simulink library "thermochemical"  (R2017b)
settings: Solver=VariableStepAuto  StartTime=0.0  StopTime=10.0  RelTol=1e-3
values from neighbouring files (symbols this model uses):
  c = conversion_factors()    [blk_clausius_clapeyron.m]    (also in blk_clausius_clapeyron_no_popup.m; blk_cold_room_closed_dry_air.m; blk_reactor_BaCl2_NH3_no_walls.m; blk_reactor_BaCl2_NH3_no_walls_state_space.m)
  cp = metal.cp    [blk_wall_simple.m]    (also in get_metal_properties.m = 390)
  fluid = get_param(blk,'fluid')    [blk_thermodynamic_properties_nonsaturated.m]    (also in blk_thermodynamic_properties_nonsaturated_interpreted.m; blk_thermodynamic_properties_saturated.m; blk_thermodynamic_properties_saturated_interpreted.m; blk_thermodynamic_properties_saturated_mix.m)
  gas = get_material_properties(x.gasName)    [blk_reactor_BaCl2_NH3_cylindrical_no_walls_fun1.m]
  h = get_param(gcb,'ObjectParameters')    [get_param_eval.m]
  rho = metal.rho    [blk_wall_simple.m]    (also in get_metal_properties.m = 8940)
  s = solve(eq,dx,'ReturnConditions',true)    [LMTD_inv.m]    (also in blk_wall_simple.m = get_param_eval(blk,'s'))
  u_gas_at_T_ref = -R * T_ref    [blk_reactor_BaCl2_NH3_no_walls.m]    (also in blk_reactor_BaCl2_NH3_no_walls_state_space.m)
undefined symbols (not defined in the file or in its folder): b_motor, BaCl2, beta, CoolProp, cP_binder, cP_gas, cP_s0, cv, dh_r_0, ENG, heat_exchanger_epsilonNTU_inv_simulink, heat_exchanger_epsilonNTU_simulink, J_motor, K_cin, kappa, Km_motor, La_motor, lookup2D_BreakPoint2, M_binder, N_binder, N_gas_free_volume_init, N_salt, NH3, nh3_v3, nu, P, phase, PID_D_motor, PID_I_motor, PID_P_motor, Ra_motor, Reactor_phase, T, T1, T2, T_init, Tr_init, Tr_ref, U_binder_at_Tr_ref, U_salt_at_X0_Tr_ref, Ur_init, V_void, Valve_regime, Vmax_motor, w_init_motor, X_init
libraries: thermochemical x247, simulink x54, dspsigops x3
(part 1 of 12)
settings Model: Creator=ferru  LastModifiedBy=fferrucc

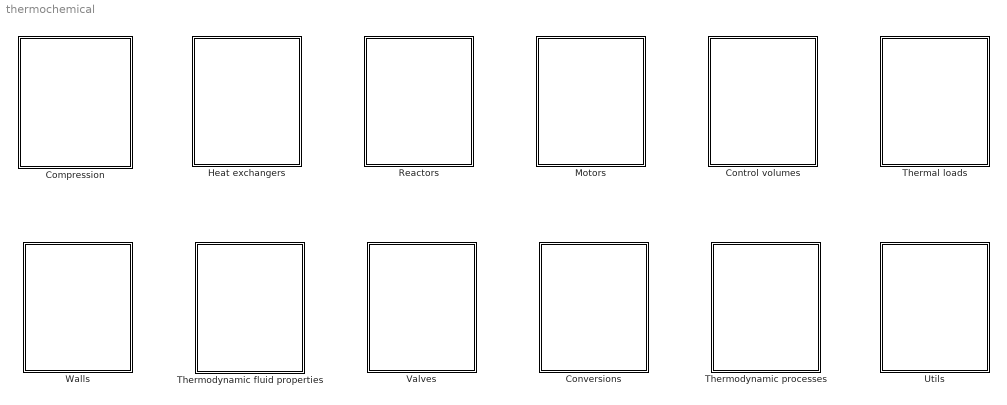
== system thermochemical ==
  Compression : Subsystem
  Control volumes : Subsystem
  Conversions : Subsystem
  Heat exchangers : Subsystem
  Motors : Subsystem
  Reactors : Subsystem
  Thermal loads : Subsystem
  Thermodynamic fluid properties : Subsystem
  Thermodynamic processes : Subsystem
  Utils : Subsystem
  Valves : Subsystem
  Walls : Subsystem

== system thermochemical/Compression ==
  Gas compressor without motor : Subsystem  mask{fluid=fluid, eta_IS=0.7, CL=0.03, eta_mech=0.9, dVswept_m3_h=6, dVswept_rmp=1500}
      mask prompts: fluid "Fluid properties (structure data type)"; eta_IS "Isentropic efficiency ([0..1])"; CL "Cylinder clearance ([0..1])"; eta_mech "Mechanical efficiency (compressor without motor) ([0..1])"; dVswept_m3_h "Swept volume rate at nominal speed (m³/h)"; dVswept_rmp "Nominal speed (rpm)"
      mask init:
      | % bar to Pascal conversion:
      | bar_to_Pa = 1e5;
  "Gas compressor without motor, two stages, ideal compression ratios" : Subsystem  mask{fluid=fluid, eta_IS=0.7, CL=0.03, eta_mech=0.9, dVswept_m3_h=6, dVswept_rmp=1500}
      mask prompts: fluid "Fluid properties (structure data type)"; eta_IS "Isentropic efficiency ([0..1])"; CL "Cylinder clearance ([0..1])"; eta_mech "Mechanical efficiency (compressor without motor) ([0..1])"; dVswept_m3_h "Swept volume rate at nominal speed (m³/h)"; dVswept_rmp "Nominal speed (rpm)"
      mask init:
      | % bar to Pascal conversion:
      | bar_to_Pa = 1e5;
  Irreversible compression process : Subsystem  mask(compression_irrev){fluid=fluid}
      mask prompts: fluid "Thermodynamic properties data (struct variable)"
      mask help: Irreversible compression process.
  Volumetric efficiency : Subsystem  mask(compression_volumetric_efficiency){}
      mask help:
      | Volumetric efficiency of a compression process.
      |
      | Ref: COMPRESSOR HANDBOOK, Paul C. Hanlon (editor), McGRAW-HILL, ISBN 0-07-026005-2, Sec. 1.2.5, page 1.11

== system thermochemical/Control volumes ==
  "Two-phase saturated fluid control volume (with wall, simple)" : Subsystem
  "Two-phase saturated fluid control volume (with wall, simple) (without algebraic loop)" : Subsystem
  "Two-phase saturated fluid control volume (with wall, tube with/without fins)" : Subsystem
  "Two-phase saturated fluid control volume (with wall, tube with/without fins) (without algebraic loop)" : Subsystem
  Two-phase saturated fluid control volume (without walls) : Subsystem  mask(volume_control_saturated){N_init=100, T_init=300, fluid=fluid, V=0.01}
      mask prompts: N_init "Initial number of mols inside the control volume (mol)"; T_init "Fluid initial temperature (K)"; fluid "Fluid (structure data type)"; V "Volume (m3)"
      mask help:
      | This block models a volume control that contains a fluid always in its saturation state.
      |
      | The model can work as a condenser or as an evaporator:
      | • Condenser: connect the output 'h liq (J/mol)' to the input 'h out (sat) (J/mol)'
      | • Evaporator: connect the output 'h vap (J/mol)' to the input 'h out (sat) (J/mol)'
      |
      | The ratio between the two phases is given by two outputs:
      | 1) volumetric liquid fraction: liquid volume/total volume (0..1)
      | 2) vapor quality (e.g. zero: 100% liquid, one: 100% vapor).
      |
      | Note 2: the model is not prepared to work in the non-saturation state of the fluid (e.g. superheated gas or supercooled liquid). This means that both the liquid fraction and the vapor quality are strictly constrained in the (0..1) open range. The simulation will stop if these constrains are violated.
      mask DialogControl Container3 Prompt: Initial state
      mask DialogControl Container4 Prompt: Other parameters
  Two-phase saturated fluid control volume (without walls) (without algebraic loop) : Subsystem  mask(volume_control_saturated){N_init=100, T_init=300, fluid=fluid, V=0.01}
      mask prompts: N_init "Initial number of mols inside the control volume (mol)"; T_init "Fluid initial temperature (K)"; fluid "Fluid (structure data type)"; V "Volume (m3)"
      mask help:
      | This block models a volume control that contains a fluid always in its saturation state.
      |
      | The model can work as a condenser or as an evaporator:
      | • Condenser: connect the output 'h liq (J/mol)' to the input 'h out (sat) (J/mol)'
      | • Evaporator: connect the output 'h vap (J/mol)' to the input 'h out (sat) (J/mol)'
      |
      | The ratio between the two phases is given by two outputs:
      | 1) volumetric liquid fraction: liquid volume/total volume (0..1)
      | 2) vapor quality (e.g. zero: 100% liquid, one: 100% vapor).
      |
      | Note 2: the model is not prepared to work in the non-saturation state of the fluid (e.g. superheated gas or supercooled liquid). This means that both the liquid fraction and the vapor quality are strictly constrained in the (0..1) open range. The simulation will stop if these constrains are violated.
      mask init:
      | c = conversion_factors();
      mask DialogControl Container3 Prompt: Initial state
      mask DialogControl Container4 Prompt: Other parameters
  Two-phase saturated fluid control volume energy equation : Subsystem  mask(control_volume_energy_equation){fluid=fluid}
      mask prompts: fluid "Fluid (structure data type)"
  "Two-phase saturated fluid control volume (with wall, simple) + heat exchanger (condensation/evaporation), with water loop" : Subsystem
  "Two-phase saturated fluid control volume (with wall, simple) + heat exchanger (condensation/evaporation), with water loop (without algebraic loop)" : Subsystem

== system thermochemical/Conversions ==
  Pressure conversion : Subsystem  mask(convert_pressure){sel=Pa --> bar}
      mask prompts: sel "Conversion"
      mask help: Conversion between pressure units.
      mask init:
      | % Get mask parameters:
      | blk = gcb;
      | par = get_param(blk,'sel');
      | c = conversion_factors();
      | switch par
      | %-----------------
      |     case 'Pa --> bar'
      |         in1    = '(Pa)';
      |         out1   = '(bar)';
      |         K = c.Pa_to_bar;
      |     case 'Pa --> kPa'
      |         in1    = '(Pa)';
      |         out1   = '(kPa)';
      |         K = c.Pa_to_kPa;
      |     case 'Pa --> psi'
      |         in1   = '(Pa)';
      |         out1  = '(psi)';
      |         K = c.Pa_to_psi;
      |     case 'Pa --> atm'
      |         in1    = '(Pa)';
      |         out1   = '(atm)';
      |         K = c.Pa_to_atm;
      | %-----------------
      |     case 'kPa --> bar'
      |         in1    = '(kPa)';
      |         out1   = '(bar)';
      |         K = c.kPa_to_bar;
      |     case 'kPa --> Pa'
      |         in1    = '(kPa)';
      |         out1   = '(Pa)';
      |         K = c.kPa_to_Pa;
      |     case 'kPa --> psi'
      |         in1   = '(kPa)';
      |         out1  = '(psi)';
      |         K = c.kPa_to_psi;
      |     case 'kPa --> atm'
      |         in1    = '(kPa)';
      |         out1   = '(atm)';
      |         K = c.kPa_to_atm;
      | %-----------------
      |     case 'bar --> Pa'
      |         in1    = '(bar)';
      |         out1   = '(Pa)';
      |         K = c.bar_to_Pa;
      |     case 'bar --> kPa'
      |         in1    = '(bar)';
      |         out1   = '(kPa)';
      |         K = c.bar_to_kPa;
      |     case 'bar --> psi'
      |         in1   = '(bar)';
      |         out1  = '(psi)';
      |         K = c.bar_to_psi;
      |     case 'bar --> atm'
      |         in1    = '(bar)';
      |         out1   = '(atm)';
      |         K = c.bar_to_atm;
      | %-----------------      
      |     case 'psi --> bar'
      |         in1   = '(psi)';
      |         out1  = '(bar)';
      |         K = c.psi_to_bar;
      |     case 'psi --> Pa'
      |         in1    = '(psi)';
      |         out1   = '(Pa)';
      |         K = c.psi_to_Pa;
      |     case 'psi --> kPa'
      |         in1    = '(psi)';
      |         out1   = '(kPa)';
      |         K = c.psi_to_kPa;
      |     case 'psi --> atm'
      |         in1    = '(psi)';
      |         out1   = '(atm)';
      |         K = c.psi_to_atm;
      | %-----------------
      |     case 'atm --> bar'
      |         in1   = '(atm)';
      |         out1  = '(bar)';
      |         K = c.atm_to_bar;
      |     case 'atm --> Pa'
      |         in1    = '(atm)';
      |         out1   = '(Pa)';
      |         K = c.atm_to_Pa;
      |     case 'atm --> kPa'
      |         in1    = '(atm)';
      |         out1   = '(kPa)';
      |         K = c.atm_to_kPa;
      |     case 'atm --> psi'
      |         in1   = '(atm)';
      |         out1  = '(psi)';
      |         K = c.atm_to_psi;
      | %-----------------
      | end
      | 
      | % % Set mask parameters:
      | set_param([blk,'/Gain'],'Gain',num2str(K))
      | % 
      | % % Change name of input 1:
      | p = get_param([blk,'/In1'],'PortHandles');
      | q = get_param(p.Outport,'Line');
      | set_param(q,'Name',in1);
      | % 
      | % % Change name of output:
      | p = get_param([blk,'/Out1'],'PortHandles');
      | q = get_param(p.Inport,'Line');
      | set_param(q,'Name',out1);
      mask TypeOptions sel: Pa --> bar | Pa --> kPa | Pa --> psi | Pa --> atm | kPa --> bar | kPa --> Pa | kPa --> psi | kPa --> atm | bar --> Pa | bar --> kPa | bar --> psi | bar --> atm | psi --> bar | psi --> Pa | psi --> kPa | psi --> atm | atm --> bar | atm --> Pa | atm --> kPa | atm --> psi
  Rotational speed conversion : Subsystem  mask(convert_pressure){sel=rpm --> rad/sec}
      mask prompts: sel "Conversion"
      mask help: Conversion between pressure units.
      mask init:
      | % Get mask parameters:
      | blk = gcb;
      | par = get_param(blk,'sel');
      | c = conversion_factors();
      | 
      | switch par
      | %-----------------
      |     case 'rpm --> rad/sec'
      |         in1    = '(rpm)';
      |         out1   = '(rad/sec)';
      |         K = c.rpm_to_rad_sec;
      |     case 'rpm --> rev/sec'
      |         in1    = '(rpm)';
      |         out1   = '(rev/sec)';
      |         K = c.rpm_to_rev_sec;
      |     case 'rad/sec --> rpm'
      |         in1   = '(rad/sec)';
      |         out1  = '(rpm)';
      |         K = c.rad_sec_to_rpm;
      |     case 'rad/sec --> rev/sec'
      |         in1    = '(rad/sec)';
      |         out1   = '(rev/sec)';
      |         K = c.rad_sec_to_rev_sec;
      |     case 'rev/sec --> rpm'
      |         in1    = '(rev/sec)';
      |         out1   = '(rpm)';
      |         K = c.rev_sec_to_rpm;
      |     case 'rev/sec --> rad/sec'
      |         in1    = '(rev/sec)';
      |         out1   = '(rad/sec)';
      |         K = c.rev_sec_to_rad_sec;
      |     otherwise
      |         error('It shouldn''t have gotten in her!')
      | end
      | 
      | % % Set mask parameters:
      | set_param([blk,'/Gain'],'Gain',num2str(K))
      | % 
      | % % Change name of input 1:
      | p = get_param([blk,'/In1'],'PortHandles');
      | q = get_param(p.Outport,'Line');
      | set_param(q,'Name',in1);
      | % 
      | % % Change name of output:
      | p = get_param([blk,'/Out1'],'PortHandles');
      | q = get_param(p.Inport,'Line');
      | set_param(q,'Name',out1);
      mask TypeOptions sel: rpm --> rad/sec | rpm --> rev/sec | rad/sec --> rpm | rad/sec --> rev/sec | rev/sec --> rpm | rev/sec --> rad/sec
  Temperature conversion : Subsystem  mask(convert_temperature){sel=°R --> °F}
      mask prompts: sel "Conversion"
      mask help: Conversion between temperature units.
      mask init:
      | % Get mask parameters:
      | blk = gcb;
      | par = get_param(blk,'sel');
      | 
      | switch par
      |     case 'K --> °C'
      |         in1   = '(K)';
      |         out1  = '(°C)';
      |         count = 1;
      |     case '°C --> K'
      |         in1   = '(°C)';
      |         out1  = '(K)';
      |         count = 2;
      |     case '°C --> °F'
      |         in1   = '(°C)';
      |         out1  = '(°F)';
      |         count = 3;  
      |     case '°F --> °C'
      |         in1    = '(°F)';
      |         out1   = '(°C)';
      |         count = 4;     
      |     case 'K --> °F'
      |         in1   = '(K)';
      |         out1  = '(°F)';
      |         count = 5;
      |     case '°F --> K'
      |         in1    = '(°F)';
      |         out1  = '(K)';
      |         count = 6;
      |     case '°R --> °C'
      |         in1   = '(°R)';
      |         out1  = '(°C)';
      |         count = 7;
      |     case '°C --> °R'
      |         in1   = '(°C)';
      |         out1  = '(°R)';
      |         count = 8;
      |     case '°R --> °F'
      |         in1   = '(°R)';
      |         out1  = '(°F)';
      |         count = 9;  
      |     case '°F --> °R'
      |         in1    = '(°F)';
      |         out1   = '(°R)';
      |         count = 10;
      |     case 'K --> °R'
      |         in1   = '(K)';
      |         out1  = '(°R)';
      |         count = 11;
      |     case '°R --> K'
      |         in1    = '(°R)';
      |         out1  = '(K)';
      |         count = 12;
      | end
      | 
      | % Set mask parameters:
      | set_param([blk,'/Constant'],'Value',num2str(count))
      | 
      | % Change name of input 1:
      | p = get_param([blk,'/In1'],'PortHandles');
      | q = get_param(p.Outport,'Line');
      | set_param(q,'Name',in1);
      | 
      | % Change name of output:
      | p = get_param([blk,'/Out1'],'PortHandles');
      | q = get_param(p.Inport,'Line');
      | set_param(q,'Name',out1);
      mask TypeOptions sel: K --> °C | K --> °F | K --> °R | °C --> K | °C --> °F | °C --> °R | °F --> K | °F --> °C | °F --> °R | °R --> K | °R --> °C | °R --> °F
  Volume flow rate conversion : Subsystem  mask(convert_volume_flow){sel=m3/h --> CFM}
      mask prompts: sel "Conversion"
      mask help: Conversion between volume flow rate units.
      mask init:
      | % Get mask parameters:
      | blk = gcb;
      | par = get_param(blk,'sel');
      | c = conversion_factors();
      | 
      | switch par
      |     case 'm3/sec --> m3/h'
      |         in1    = '(m3/sec)';
      |         out1   = '(m3/h)';    
      |         K      = c.m3_sec_to_m3_h;
      |     case 'm3/sec --> L/min'
      |         in1    = '(m3/sec)';
      |         out1   = '(L/min)';    
      |         K      = c.m3_sec_to_L_min;
      |     case 'm3/sec --> gpmUS'
      |         in1    = '(m3/sec)';
      |         out1   = '(gpmUS)';    
      |         K      = c.m3_sec_to_gpmUS;
      |     case 'm3/sec --> CFH'
      |         in1    = '(m3/sec)';
      |         out1   = '(CFH)';    
      |         K      = c.m3_sec_to_CFH;
      |     case 'm3/sec --> CFM'
      |         in1    = '(m3/sec)';
      |         out1   = '(CFM)';    
      |         K      = c.m3_sec_to_CFM;
      |     case 'L/min --> m3/sec'
      |         in1    = '(L/min)';
      |         out1   = '(m3/sec)';    
      |         K      = c.L_min_to_m3_sec;
      |     case 'L/min --> m3/h'
      |         in1    = '(L/min)';
      |         out1   = '(m3/h)';    
      |         K      = c.L_min_to_m3_h;
      |     case 'L/min --> gpmUS'
      |         in1    = '(L/min)';
      |         out1   = '(gpmUS)';    
      |         K      = c.L_min_to_gpmUS;
      |     case 'L/min --> CFH'
      |         in1    = '(L/min)';
      |         out1   = '(CFH)';    
      |         K      = c.L_min_to_CFH;
      |     case 'L/min --> CFM'
      |         in1    = '(L/min)';
      |         out1   = '(CFM)';    
      |         K      = c.L_min_to_CFM;
      |     case 'm3/h --> m3/sec'
      |         in1    = '(m3/h)';
      |         out1   = '(m3/sec)';    
      |         K      = c.m3_h_to_m3_sec;
      |     case 'm3/h --> L/min'
      |         in1    = '(m3/h)';
      |         out1   = '(L/min)';    
      |         K      = c.m3_h_to_L_min;
      |     case 'm3/h --> gpmUS'
      |         in1    = '(m3/h)';
      |         out1   = '(gpmUS)';    
      |         K      = c.m3_h_to_gpmUS;
      |     case 'm3/h --> CFH'
      |         in1    = '(m3/h)';
      |         out1   = '(CFH)';    
      |         K      = c.m3_h_to_CFH;
      |     case 'm3/h --> CFM'
      |         in1    = '(m3/h)';
      |         out1   = '(CFM)';    
      |         K      = c.m3_h_to_CFM;
      |     case 'gpmUS --> m3/sec'
      |         in1    = '(gpmUS)';
      |         out1   = '(m3/sec)';    
      |         K      = c.gpmUS_to_m3_sec;
      |     case 'gpmUS --> m3/h'
      |         in1    = '(gpmUS)';
      |         out1   = '(m3/h)';    
      |         K      = c.gpmUS_to_m3_h;
      |     case 'gpmUS --> L/min'
      |         in1    = '(gpmUS)';
      |         out1   = '(L/min)';    
      |         K      = c.gpmUS_to_L_min;
      |     case 'gpmUS --> CFH'
      |         in1    = '(gpmUS)';
      |         out1   = '(CFH)';    
      |         K      = c.gpmUS_to_CFH;
      |     case 'gpmUS --> CFM'
      |         in1    = '(gpmUS)';
      |         out1   = '(CFM)';    
      |         K      = c.gpmUS_to_CFM;
      |     case 'CFH --> m3/sec'
      |         in1    = '(CFH)';
      |         out1   = '(m3/sec)';    
      |         K      = c.CFH_to_m3_sec;
      |     case 'CFH --> m3/h'
      |         in1    = '(CFH)';
      |         out1   = '(m3/h)';    
      |         K      = c.CFH_to_m3_h;
      |     case 'CFH --> L/min'
      |         in1    = '(CFH)';
      |         out1   = '(L/min)';    
      |         K      = c.CFH_to_L_min;
      |     case 'CFH --> gpmUS'
      |         in1    = '(CFH)';
      |         out1   = '(gpmUS)';    
      |         K      = c.CFH_to_gpmUS;
      |     case 'CFH --> CFM'
      |         in1    = '(CFH)';
      |         out1   = '(CFM)';    
      |         K      = c.CFH_to_CFM;
      |     case 'CFM --> m3/sec'
      |         in1    = '(CFM)';
      |         out1   = '(m3/sec)';    
      |         K      = c.CFM_to_m3_sec;
      |     case 'CFM --> m3/h'
      |         in1    = '(CFM)';
      |         out1   = '(m3/h)';    
      |         K      = c.CFM_to_m3_h;
      |     case 'CFM --> L/min'
      |         in1    = '(CFM)';
      |         out1   = '(L/min)';    
      |         K      = c.CFM_to_L_min;
      |     case 'CFM --> gpmUS'
      |         in1    = '(CFM)';
      |         out1   = '(gpmUS)';    
      |         K      = c.CFM_to_gpmUS;
      |     case 'CFM --> CFH'
      |         in1    = '(CFM)';
      |         out1   = '(CFH)';    
      |         K      = c.CFM_to_CFH;
      |     otherwise
      |         error('It shouldn''t have entered here!')
      | end
      | 
      | % Set mask parameters:
      | set_param([blk,'/Gain'],'Gain',num2str(K))
      |  
      | % Change name of input 1:
      | p = get_param([blk,'/In1'],'PortHandles');
      | q = get_param(p.Outport,'Line');
      | set_param(q,'Name',in1);
      |  
      | % Change name of output:
      | p = get_param([blk,'/Out1'],'PortHandles');
      | q = get_param(p.Inport,'Line');
      | set_param(q,'Name',out1);
      mask TypeOptions sel: m3/sec --> m3/h | m3/sec --> L/min | m3/sec --> gpmUS | m3/sec --> CFH | m3/sec --> CFM | L/min --> m3/sec | L/min --> m3/h | L/min --> gpmUS | L/min --> CFH | L/min --> CFM | m3/h --> m3/sec | m3/h --> L/min | m3/h --> gpmUS | m3/h --> CFH | m3/h --> CFM | gpmUS --> m3/sec | gpmUS --> m3/h | gpmUS --> L/min | gpmUS --> CFH | gpmUS --> CFM | CFH --> m3/sec | CFH --> m3/h | CFH --> L/min | CFH --> gpmUS | CFH --> CFM | CFM --> m3/sec | CFM --> m3/h | CFM --> L/min | CFM --> gpmUS | CFM --> CFH

== system thermochemical/Heat exchangers ==
  "Heat Exchanger, e-NTU method (UA input) (it uses CoolProp library)" : Subsystem  mask(heat_exchanger_eNTU){fluidName_1=Water, fluidName_2=Water, flowType=Counter-flow}
      mask prompts: fluidName_1 "Stream 1 fluid name (must be available in CoolProp library)"; fluidName_2 "Stream 2 fluid name (must be available in CoolProp library)"; flowType "Flow arrangement"
      mask help:
      | Heat Exchanger, e-NTU method.
      | The block assumes:
      | * null pressure drop in the streams
      | * steady state
      | The values of heat capacities are computed at an average temperature value between the inlet and outlet temperatures. The block uses the CoolProp library (see help for references).
      |
      | The dimensionless number Cr = d(Cmin)/dt / d(Cmax)/dt is the capacity ratio and reﬂects how well-balanced the heat exchanger is.
      | If the capacity ratio is unity, then the heat exchanger is operating in a balanced condition; the capacitance rates of the two ﬂuids and therefore the temperature change experienced by the two ﬂuids are the same. If the capacity ratio is very small, then the heat exchanger is operating in an unbalanced condition; the capacitance rate of one ﬂuid is very large compared to the other and the temperature of this ﬂuid will not change substantially. This situation occurs when one ﬂuid is changing phase.
      mask init:
      | % NOTE: Everything that is writen here will go to MaskInitialization parameter
      | 
      | % Get mask parameters:
      | blk = gcb;
      | fluidName_h = get_param(blk,'fluidName_1');
      | fluidName_c = get_param(blk,'fluidName_2');
      | flowType = get_param(blk,'flowType');
      | 
      | % Set value of Interpreted Matlab function according to menu's parameters:
      | str = ['heat_exchanger_epsilonNTU_simulink(u(1),u(2),u(3),''',fluidName_1,''',u(4),u(5),u(6),''',fluidName_2,''',u(7),''',flowType,''')'];
      | set_param([blk,'/heat_exchanger'],'MATLABFcn',str);
      | 
      | % Debug only:
      | % disp(str)
      mask Help:
      | Ref:
      | [1] Gregory Nellis, Sanford Klein -  Heat Transfer - Cambridge University Press (2008). Section 8.
      | [2] Ian H. Bell, Jorrit Wronski, Sylvain Quoilin, and Vincent Lemort,Pure and pseudo-pure fluid thermophysical  property evaluation  and  the  open-source  thermophysical  property  library  cool-prop, Industrial & Engineering Chemistry Research 53 (2014), no. 6, 2498–2508.
      mask TypeOptions flowType: Counter-flow | Parallel-flow | Cross-flow, both unmixed | Cross-flow, both mixed | Cross-flow, Cmax mixed, Cmin unmixed | Cross-flow, Cmin mixed, Cmax unmixed
  "Heat Exchanger, e-NTU method (UA input) Loop 2: water" : Subsystem  mask(heat_exchanger_eNTU_inv_2){fluid=fluid, flowType=Counter-flow, cp_water_J_K_mol=75.3260}
      mask prompts: fluid "Thermodynamic properties data for fluid 1 (struct variable)"; flowType "Flow arrangement"; cp_water_J_K_mol "Cp of water (J/K·mol)"
      mask help:
      | Heat Exchanger, e-NTU method (inverse)
      | The block accepts 'epsilon' as input and returns the conductance 'U*A' (W/K).
      | The block assumes:
      | * null pressure drop in the streams
      | * steady state
      | * loop 2 fluid is water
      | The values of heat capacity for fluid in loop 1 is computed at an average temperature value between the inlet and outlet temperatures.
      |
      | The dimensionless number Cr = d(Cmin)/dt / d(Cmax)/dt is the capacity ratio and reﬂects how well-balanced the heat exchanger is.
      | If the capacity ratio is unity, then the heat exchanger is operating in a balanced condition; the capacitance rates of the two ﬂuids and therefore the temperature change experienced by the two ﬂuids are the same. If the capacity ratio is very small, then the heat exchanger is operating in an unbalanced condition; the capacitance rate of one ﬂuid is very large compared to the other and the temperature of this ﬂuid will not change substantially. This situation occurs when one ﬂuid is changing phase.
      mask init:
      | % NOTE: Everything that is writen here will go to MaskInitialization parameter
      | 
      | % Get mask parameters:
      | blk = gcb;
      | flow = get_param(blk,'flowType');
      | 
      | % Compute 'flowType_numeric' according to 'flowType' dialog variable:
      | switch(flow)
      |     case 'Counter-flow'
      |         flowType_numeric = 0;
      |     case 'Parallel-flow'
      |         flowType_numeric = 1;
      |     case 'Cross-flow, both unmixed'
      |         flowType_numeric = 2;
      |     case 'Cross-flow, both mixed'
      |         flowType_numeric = 3;
      |     case 'Cross-flow, Cmax mixed, Cmin unmixed'
      |         flowType_numeric = 4;
      |     case 'Cross-flow, Cmin mixed, Cmax unmixed'
      |         flowType_numeric = 5;
      |     case 'Condensation/evaporation'
      |         flowType_numeric = 6;
      |     otherwise
      |         flowType_numeric = -1;
      |         error('Wrong flow type or flow type not implemented.')
      | end
      | 
      | % Set value of constant block:
      | set_param([blk,'/Subsystem/NTU as a function of flow configuration/Flow type (numeric)'],...
      |            'Value',num2str(flowType_numeric));
      mask Help:
      | Ref:
      | [1] Gregory Nellis, Sanford Klein -  Heat Transfer - Cambridge University Press (2008). Section 8.
      | [2] Ian H. Bell, Jorrit Wronski, Sylvain Quoilin, and Vincent Lemort,Pure and pseudo-pure fluid thermophysical  property evaluation  and  the  open-source  thermophysical  property  library  cool-prop, Industrial & Engineering Chemistry Research 53 (2014), no. 6, 2498–2508.
      mask TypeOptions flowType: Counter-flow | Parallel-flow | Cross-flow, both unmixed | Cross-flow, Cmax mixed, Cmin unmixed | Cross-flow, Cmin mixed, Cmax unmixed
  "Heat Exchanger, e-NTU method (UA input) One fluid or condensation/evaporation Loop 2: water" : Subsystem  mask(heat_exchanger_one_fluid_eNTU){cp_water_J_K_mol=75.3260}
      mask prompts: cp_water_J_K_mol "Cp of water (J/K·mol)"
      mask help:
      | Heat Exchanger, one-fluid configuration (isothermal wall), e-NTU method
      |
      | The block accepts the conductance 'U*A' (W/K) as input and returns 'epsilon'.
      |
      | The block assumes:
      | * null pressure drop in the water stream
      | * steady state
      | * loop 1 has constant temperature
      | * loop 2 fluid is water
      mask Help:
      | Ref:
      | [1] Gregory Nellis, Sanford Klein -  Heat Transfer - Cambridge University Press (2008). Section 8.
      | [2] Ian H. Bell, Jorrit Wronski, Sylvain Quoilin, and Vincent Lemort,Pure and pseudo-pure fluid thermophysical  property evaluation  and  the  open-source  thermophysical  property  library  cool-prop, Industrial & Engineering Chemistry Research 53 (2014), no. 6, 2498–2508.
  "Heat Exchanger, e-NTU method (epsilon input) (it uses CoolProp library)" : Subsystem  mask(heat_exchanger_eNTU_inv){fluidName_1=Water, fluidName_2=Water, flowType=Counter-flow}
      mask prompts: fluidName_1 "Stream 1 fluid name (must be available in CoolProp library)"; fluidName_2 "Stream 2 fluid name (must be available in CoolProp library)"; flowType "Flow arrangement"
      mask help:
      | Heat Exchanger, e-NTU method (inverse)
      | The block accepts 'epsilon' as input and returns the conductance 'U*A' (W/K).
      | The block assumes:
      | * null pressure drop in the streams
      | * steady state
      | The values of heat capacities are computed at an average temperature value between the inlet and outlet temperatures. The block uses the CoolProp library (see help for references).
      |
      | The dimensionless number Cr = d(Cmin)/dt / d(Cmax)/dt is the capacity ratio and reﬂects how well-balanced the heat exchanger is.
      | If the capacity ratio is unity, then the heat exchanger is operating in a balanced condition; the capacitance rates of the two ﬂuids and therefore the temperature change experienced by the two ﬂuids are the same. If the capacity ratio is very small, then the heat exchanger is operating in an unbalanced condition; the capacitance rate of one ﬂuid is very large compared to the other and the temperature of this ﬂuid will not change substantially. This situation occurs when one ﬂuid is changing phase.
      mask init:
      | % NOTE: Everything that is writen here will go to MaskInitialization parameter
      | 
      | % Get mask parameters:
      | blk = gcb;
      | fluidName_1 = get_param(blk,'fluidName_1');
      | fluidName_2 = get_param(blk,'fluidName_2');
      | flowType = get_param(blk,'flowType');
      | 
      | % Set value of Interpreted Matlab function according to menu's parameters:
      | str = ['heat_exchanger_epsilonNTU_inv_simulink(u(1),u(2),u(3),''',fluidName_1,''',u(4),u(5),u(6),''',fluidName_2,''',u(7),''',flowType,''')'];
      | set_param([blk,'/heat_exchanger'],'MATLABFcn',str);
      | 
      | % Debug only:
      | % disp(str)
      mask Help:
      | Ref:
      | [1] Gregory Nellis, Sanford Klein -  Heat Transfer - Cambridge University Press (2008). Section 8.
      | [2] Ian H. Bell, Jorrit Wronski, Sylvain Quoilin, and Vincent Lemort,Pure and pseudo-pure fluid thermophysical  property evaluation  and  the  open-source  thermophysical  property  library  cool-prop, Industrial & Engineering Chemistry Research 53 (2014), no. 6, 2498–2508.
      mask TypeOptions flowType: Counter-flow | Parallel-flow | Cross-flow, both unmixed | Cross-flow, Cmax mixed, Cmin unmixed | Cross-flow, Cmin mixed, Cmax unmixed
  "Heat Exchanger, e-NTU method (epsilon input) Loop 2: water" : Subsystem  mask(heat_exchanger_eNTU_inv_2){fluid=fluid, flowType=Counter-flow, cp_water_J_K_mol=75.3260}
      mask prompts: fluid "Thermodynamic properties data for fluid 1 (struct variable)"; flowType "Flow arrangement"; cp_water_J_K_mol "Cp of water (J/K·mol)"
      mask help:
      | Heat Exchanger, e-NTU method (inverse)
      | The block accepts 'epsilon' as input and returns the conductance 'U*A' (W/K).
      | The block assumes:
      | * null pressure drop in the streams
      | * steady state
      | * loop 2 fluid is water
      | The values of heat capacity for fluid in loop 1 is computed at an average temperature value between the inlet and outlet temperatures.
      |
      | The dimensionless number Cr = d(Cmin)/dt / d(Cmax)/dt is the capacity ratio and reﬂects how well-balanced the heat exchanger is.
      | If the capacity ratio is unity, then the heat exchanger is operating in a balanced condition; the capacitance rates of the two ﬂuids and therefore the temperature change experienced by the two ﬂuids are the same. If the capacity ratio is very small, then the heat exchanger is operating in an unbalanced condition; the capacitance rate of one ﬂuid is very large compared to the other and the temperature of this ﬂuid will not change substantially. This situation occurs when one ﬂuid is changing phase.
      mask init: same as thermochemical/Heat exchangers/Heat Exchanger, e-NTU method (UA input) Loop 2: water
      mask Help:
      | Ref:
      | [1] Gregory Nellis, Sanford Klein -  Heat Transfer - Cambridge University Press (2008). Section 8.
      | [2] Ian H. Bell, Jorrit Wronski, Sylvain Quoilin, and Vincent Lemort,Pure and pseudo-pure fluid thermophysical  property evaluation  and  the  open-source  thermophysical  property  library  cool-prop, Industrial & Engineering Chemistry Research 53 (2014), no. 6, 2498–2508.
      mask TypeOptions flowType: Counter-flow | Parallel-flow | Cross-flow, both unmixed | Cross-flow, Cmax mixed, Cmin unmixed | Cross-flow, Cmin mixed, Cmax unmixed
  "Heat Exchanger, e-NTU method (epsilon input) One fluid or condensation/evaporation Loop 2: water" : Subsystem  mask(heat_exchanger_one_fluid_eNTU_inv){cp_water_J_K_mol=75.3260}
      mask prompts: cp_water_J_K_mol "Cp of water (J/K·mol)"
      mask help:
      | Heat Exchanger, one-fluid configuration (isothermal wall), e-NTU method (inverse)
      |
      | The block accepts 'epsilon' as input and returns the conductance 'U*A' (W/K).
      |
      | The block assumes:
      | * null pressure drop in the water stream
      | * steady state
      | * loop 1 has constant temperature
      | * loop 2 fluid is water
      mask Help:
      | Ref:
      | [1] Gregory Nellis, Sanford Klein -  Heat Transfer - Cambridge University Press (2008). Section 8.
      | [2] Ian H. Bell, Jorrit Wronski, Sylvain Quoilin, and Vincent Lemort,Pure and pseudo-pure fluid thermophysical  property evaluation  and  the  open-source  thermophysical  property  library  cool-prop, Industrial & Engineering Chemistry Research 53 (2014), no. 6, 2498–2508.
  LMTD : Subsystem

== system thermochemical/Motors ==
  DC motor + DC power supply + speed controller : Subsystem  mask(dc_motor_plus_speed_controller_plus_DC_power_source){L=La_motor, R=Ra_motor, J=J_motor, b=b_motor, Km=Km_motor, w_init_motor=w_init_motor, PID_P=PID_P_motor, PID_I=PID_I_motor, PID_D=PID_D_motor, V_max=Vmax_motor}
      mask prompts: L "Armature inductance (Hy)"; R "Armature resistance (Ohm)"; J "Mechanical inertia (kg.m²)"; b "Viscous friction coefficient (N.m.sec)"; Km "Electromechanical constant (N.m/A)"; w_init_motor "Motor initial speed (rad/sec)"; PID_P "Proportional gain"; PID_I "Integral gain"; PID_D "Derivative gain"; V_max "Maximum output voltage (V)"
      mask DialogControl Container3 Prompt: DC motor
      mask DialogControl Container4 Prompt: Motor speed controller (PDI controller)
      mask DialogControl Container5 Prompt: Power source
  "DC motor, permanent magnet, one-way rotation" : Subsystem  mask(dc_motor_permanent_magnet_one_way_rotation){L=2.31e-3, R=0.83, J=0.1, b=2.5e-4, Km=1.3, w_init=0}
      mask prompts: L "Armature inductance (Hy)"; R "Armature resistance (Ohm)"; J "Mechanical inertia (kg.m²)"; b "Viscous friction coefficient (N.m.sec)"; Km "Electromechanical constant (N.m/A)"; w_init "Motor initial speed (rad/sec)"

== system thermochemical/Reactors ==
  Reactor's internal energy equation : Subsystem  mask(reactor_internal_energy){Tr_ref=Tr_ref, N_salt=N_salt, cP_s0=cP_s0, U_salt_at_X0_Tr_ref=U_salt_at_X0_Tr_ref, N_binder=N_binder, M_binder=M_binder, cP_binder=cP_binder, U_binder_at_Tr_ref=U_binder_at_Tr_ref, V_void=V_void, gas_model_void_volume=Ideal gas model, gas_model_salt=Ideal gas model, is_ideal_gas_in_void_volume=1, is_ideal_gas_in_salt=1, fluid=fluid, cP_gas=cP_gas, u_gas_at_Tr_ref=u_gas_at_T_ref, nu=nu, dh_r=dh_r_0, R=8.314472}
      mask prompts: Tr_ref "Internal energies (salt, binder, gas) reference temperature [K]"; N_salt "Number of mols of salt [mol]"; cP_s0 "Cp of the anhydrous salt [J/(K.mol)]"; U_salt_at_X0_Tr_ref "Salt internal energy at X=0 and at reference temperature [J]"; N_binder "Number of moles binder [mol]"; M_binder "Molar mass of binder [kg/mol]"; cP_binder "Cp of binder [J/(K.kg)]"; U_binder_at_Tr_ref "Binder internal energy at reference temperature [J]"; V_void "Void volume [m³]"; gas_model_void_volume "Gas model in the void volume"; gas_model_salt "Gas model in the composite"; is_ideal_gas_in_void_volume "No need (hidden)"; is_ideal_gas_in_salt "No need (hidden)"; fluid "Gas look-up table data structure (only needed if real gas model is selected):"; cP_gas "Cp of gas (only needed if ideal gas model is selected) ([J/K/mol]"; u_gas_at_Tr_ref "Gas specific internal energy at reference temp. (only needed if ideal gas model is selected) [J/mol]"; nu "Reaction stoichiometric coefficient [mol gas/mol salt]"; dh_r "Solid/gas enthalpy of reaction [J/mol]"; R "Universal gas constant [J/K/mol]"
      mask help: Reactor's internal energy equation
      mask init:
      | % Get mask parameters:
      | blk = gcb;
      | gas_void = get_param(blk,'gas_model_void_volume');
      | gas_salt = get_param(blk,'gas_model_salt');
      | 
      | % Set variable according to parameter
      | switch gas_void
      |     case 'Ideal gas model'
      |         is_ideal_gas_void_volume = '1';
      |     case 'Real gas model'
      |         is_ideal_gas_void_volume = '-1';
      |     otherwise 
      |         error('An error occurred in the mask radio button')
      | end
      | 
      | switch gas_salt
      |     case 'Ideal gas model'
      |         is_ideal_gas_salt = '1';
      |     case 'Real gas model'
      |         is_ideal_gas_salt = '-1';
      |     otherwise 
      |         error('An error occurred in the mask radio button')
      | end
      | 
      | % Set parameter
      | set_param(blk,'is_ideal_gas_in_void_volume',is_ideal_gas_void_volume);
      | set_param(blk,'is_ideal_gas_in_salt',is_ideal_gas_salt);
      mask TypeOptions gas_model_void_volume: Ideal gas model | Real gas model
      mask TypeOptions gas_model_salt: Ideal gas model | Real gas model
      mask DialogControl Container3 Prompt: Salt
      mask DialogControl Container4 Prompt: Binder
      mask DialogControl Container5 Prompt: Gas
      mask DialogControl Container6 Prompt: Reaction
  "Reactor, BaCl2/NH3, state-space form, [Tr, Ng, X] as state variables, no algebraic loops, ideal gas in void volume, ideal gas in salt" : Subsystem
  "Reactor, BaCl2/NH3, state-space form, [Tr, Ng, X] as state variables, no algebraic loops, real gas in void volume, ideal gas in salt" : Subsystem
  "Reactor, BaCl2/NH3, state-space form, [Tr, Ng, X] as state variables, no algebraic loops, real gas in void volume, real gas in salt" : Subsystem
  "Reactor, BaCl2/NH3, state-space form, [Ur, Ng, X] as state variables, no algebraic loops, ideal gas in void volume, ideal gas in salt" : Subsystem
  "Reactor, BaCl2/NH3, with algebraic loops, ideal gas in void volume, ideal gas in salt" : Subsystem
  "Reactor, BaCl2/NH3, with algebraic loops, real gas in void volume, ideal gas in salt" : Subsystem
  "Reactor, BaCl2/NH3, with algebraic loops, real gas in void volume, real gas in salt" : Subsystem

== system thermochemical/Thermal loads ==
  "Cold room, closed, dry air (it uses CoolProp library for initialization)" : Subsystem  mask(cold_room_closed_dry_air){L=1, W=1, H=1, U=0.25, Tinit_C=30, S=6, V=1, M=1.1647, Cv=717.9716}
      mask prompts: L "Length [m]"; W "Width [m]"; H "Height [m]"; U "Walls heat transfer coefficient [W/(m²·K)]"; Tinit_C "Room initial air temperature [°C]"; S "Total surface (m²)"; V "Volume (m³)"; M "Mass (kg)"; Cv "Cv (J/kg/K)"
      mask help:
      | The model assumes the following:
      | • Empty room.
      | • Dry air.
      | • No energy accumulation at the walls.
      | • Constant Cv (computed at 300K,1atm).
      | • There is no mass transfer (closed system).
      | • The mass of dry air is computed at 1atm and at initial temperature.
      |
      | NOTES:
      | Heat released by people for different work types:
      | • Ligth: 39W/person
      | • Medium: 150W/person
      | • Heavy: 250W/person
      mask init:
      | blk_cold_room_closed_dry_air(gcb)
